simulink model "crazyflie_ponti"  (R2018b)
settings: Solver=FixedStepDiscrete  StartTime=0.0  StopTime=25  FixedStep=0.01  RelTol=1e-3
values from neighbouring files (symbols this model uses):
  gamma = 0.98    [Jonaz.mat]
  K = [-135.279629651 -135.279629543 135.279629485 135.279629377 -135.330448309 135.330448003 135.330448111 -135.330448202 -58.4203591404 -58.4203590939 58.420359069 58.4203590225 ... (20 elements, 4x5)]    [Jonaz.mat]    (also in LQRGain.mat)
undefined symbols (not defined in the file or in its folder): DiscIntNeverNeededParam
libraries: simulink x1
settings Model: PauseTimes=7  Creator=Zrean  LastModifiedBy=Jonas
settings OptimizationCC: DefaultParameterBehavior=Inlined  UseDivisionForNetSlopeComputation=on  UseFloatMulNetSlope=on  UseSpecifiedMinMax=on  InlineInvariantSignals=on  PassReuseOutputArgsAs=Individual arguments  ZeroExternalMemoryAtStartup=off  ZeroInternalMemoryAtStartup=off  NoFixptDivByZeroProtection=on  EfficientFloat2IntCast=on  LifeSpan=1
settings DebuggingCC: AlgebraicLoopMsg=error  ParameterTunabilityLossMsg=error
settings HardwareCC: ProdBitPerPointer=32  ProdBitPerSizeT=32  ProdBitPerPtrDiffT=32  ProdLargestAtomicInteger=Long  ProdLargestAtomicFloat=Double  ProdWordSize=32  ProdHWDeviceType=ARM Compatible->ARM Cortex
settings SFSimCC: SimUseLocalCustomCode=off  MATLABDynamicMemAlloc=off
settings RTWCC: SystemTargetFile=ert.tlc  GenCodeOnly=on  TemplateMakefile=ert_default_tmf  GenerateReport=on  RTWUseLocalCustomCode=off  BuildConfiguration=Faster Runs  IncludeHyperlinkInReport=on  LaunchReport=on  GenerateTraceInfo=on  GenerateTraceReport=on  GenerateTraceReportSl=on  GenerateTraceReportSf=on  GenerateTraceReportEml=on  GenerateCodeMetricsReport=on
settings CodeAppCC: ForceParamTrailComments=on  IgnoreCustomStorageClasses=off  OperatorAnnotations=on  SimulinkDataObjDesc=on  SFDataObjDesc=on  MATLABFcnDesc=on  CustomSymbolStrGlobalVar=rt$N$M  CustomSymbolStrType=$N$M  CustomSymbolStrFcn=$N$M$F  CustomSymbolStrMacro=$N$M  InsertBlockDesc=on  StateflowObjectComments=on  MATLABSourceComments=on
settings ERTTargetCC: TargetLangStandard=C99 (ISO)  MultiwordLength=2048  CombineSignalStateStructs=on  SuppressErrorStatus=on  SupportAbsoluteTime=off  SupportNonFinite=off  SupportComplex=off  InlinedParameterPlacement=NonHierarchical  ERTCustomFileTemplate=crazyflie_wrapper.tlc  ERTFilePackagingFormat=CompactWithDataFile
settings SimscapeCC: SimscapeNormalizeSystem=off

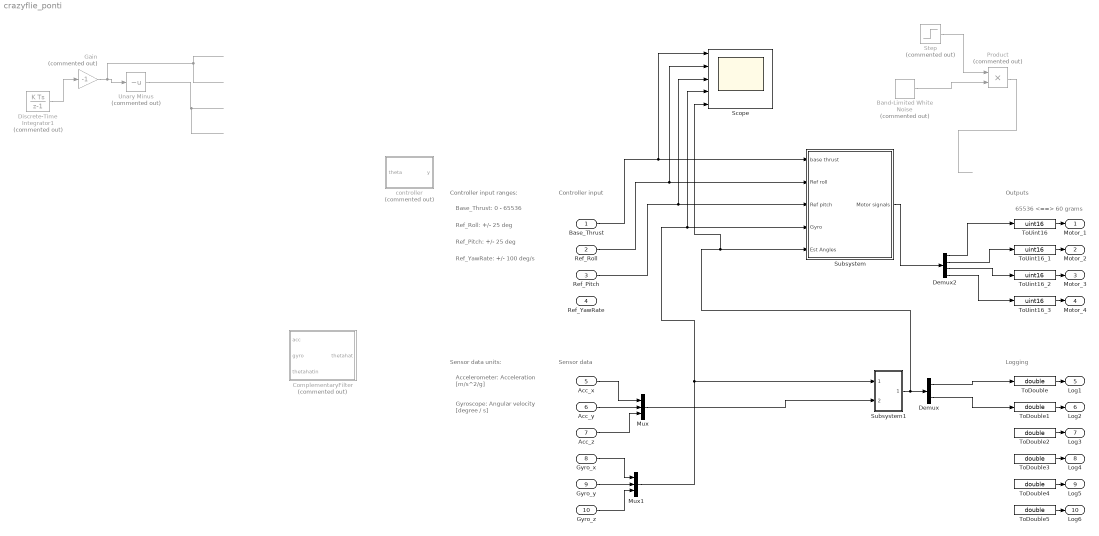
== system crazyflie_ponti ==
  note: 65536 <==> 60 grams
  note: Logging
  note: Outputs
  note: Sensor data
  note: Controller input
  note: Ref_Roll: +/- 25 deg
  note: Base_Thrust: 0 - 65536
  note: Ref_Pitch: +/- 25 deg
  note: Ref_YawRate: +/- 100 deg/s
  note: Controller input ranges:
  note: Gyroscope:
      | Angular velocity [degree / s]
  note: Accelerometer:
      | Acceleration [m/s^2/g]
  note: Sensor data units:
  Base_Thrust : Inport  OutDataTypeStr=double
  Ref_Roll : Inport  Port=2  OutDataTypeStr=double
  Ref_Pitch : Inport  Port=3  OutDataTypeStr=double
  Ref_YawRate : Inport  Port=4  OutDataTypeStr=double
  Acc_x : Inport  Port=5  OutDataTypeStr=double  PortDimensions=1
  Acc_y : Inport  Port=6  OutDataTypeStr=double  PortDimensions=1
  Acc_z : Inport  Port=7  OutDataTypeStr=double  PortDimensions=1
  Gyro_x : Inport  Port=8  OutDataTypeStr=double  PortDimensions=1
  Gyro_y : Inport  Port=9  OutDataTypeStr=double  PortDimensions=1
  Gyro_z : Inport  Port=10  OutDataTypeStr=double  PortDimensions=1
  Band-Limited White Noise : simulink/Sources/Band-Limited White Noise  Commented=on  Cov=[10]  Ts=2  seed=[23341]
  "ComplementaryFilter " : MATLAB Function  Commented=on  TreatAsAtomicUnit=on
  Demux : Demux  Outputs=2
  Demux2 : Demux
  Discrete-Time Integrator1 : DiscreteIntegrator  Commented=on  SampleTime=-1  ICPrevOutput=DiscIntNeverNeededParam  ICPrevScaledInput=DiscIntNeverNeededParam
  Gain : Gain  Commented=on  Gain=-1
  Mux : Mux  Inputs=3
  Mux1 : Mux  Inputs=3
  Product : Product  Commented=on
  Scope : Scope  NumInputPorts=5
  Step : Step  Commented=on  Time=2  After=0  SampleTime=0
  Subsystem : Subsystem
  Subsystem1 : Subsystem
  ToDouble{,1..5} (6 alike) : DataTypeConversion  OutDataTypeStr=double  SaturateOnIntegerOverflow=on
  ToUint16 : DataTypeConversion  OutDataTypeStr=uint16  SaturateOnIntegerOverflow=on
  ToUint16_1 : DataTypeConversion  OutDataTypeStr=uint16  SaturateOnIntegerOverflow=on
  ToUint16_2 : DataTypeConversion  OutDataTypeStr=uint16  SaturateOnIntegerOverflow=on
  ToUint16_3 : DataTypeConversion  OutDataTypeStr=uint16  SaturateOnIntegerOverflow=on
  Unary Minus : UnaryMinus  Commented=on
  controller : MATLAB Function  Commented=on  TreatAsAtomicUnit=on
  Motor_1 : Outport  OutDataTypeStr=uint16  LockScale=on
  Motor_2 : Outport  Port=2  OutDataTypeStr=uint16  LockScale=on
  Motor_3 : Outport  Port=3  OutDataTypeStr=uint16  LockScale=on
  Motor_4 : Outport  Port=4  OutDataTypeStr=uint16  LockScale=on
  Log1 : Outport  Port=5  OutDataTypeStr=double
  Log2 : Outport  Port=6  OutDataTypeStr=double
  Log3 : Outport  Port=7  OutDataTypeStr=double
  Log4 : Outport  Port=8  OutDataTypeStr=double
  Log5 : Outport  Port=9  OutDataTypeStr=double
  Log6 : Outport  Port=10  OutDataTypeStr=double
  wires:
  ToUint16/1 -> Motor_1/1
  ToUint16_1/1 -> Motor_2/1
  ToUint16_2/1 -> Motor_3/1
  ToUint16_3/1 -> Motor_4/1
  ToDouble/1 -> Log1/1
  ToDouble1/1 -> Log2/1
  ToDouble2/1 -> Log3/1
  ToDouble3/1 -> Log4/1
  ToDouble4/1 -> Log5/1
  ToDouble5/1 -> Log6/1
  Acc_z/1 -> Mux/3
  Acc_x/1 -> Mux/1
  Acc_y/1 -> Mux/2
  Gyro_z/1 -> Mux1/3
  Mux1/1 -> Scope/4, Subsystem/4(Gyro), Subsystem1/1(Gyro)
  Gyro_x/1 -> Mux1/1
  Gain/1 -> Unary Minus/1
  Unary Minus/1 -> ?
  Discrete-Time Integrator1/1 -> Gain/1
  Demux2/2 -> ToUint16_1/1
  Demux2/3 -> ToUint16_2/1
  Demux2/4 -> ToUint16_3/1
  Gyro_y/1 -> Mux1/2
  Base_Thrust/1 -> Scope/1, Subsystem/1(base thrust)
  Ref_Roll/1 -> Scope/2, Subsystem/2(Ref roll)
  Ref_Pitch/1 -> Scope/3, Subsystem/3(Ref pitch)
  Subsystem/1("Motor signals ") -> Demux2/1
  Mux/1 -> Subsystem1/2(Acc)
  Subsystem1/1(Out1) -> Demux/1, Scope/5, Subsystem/5(Est Angles)
  Demux2/1 -> ToUint16/1
  Step/1 -> Product/1
  Band-Limited White Noise/1 -> Product/2
  Product/1 -> ?
  Demux/1 -> ToDouble/1
  Demux/2 -> ToDouble1/1

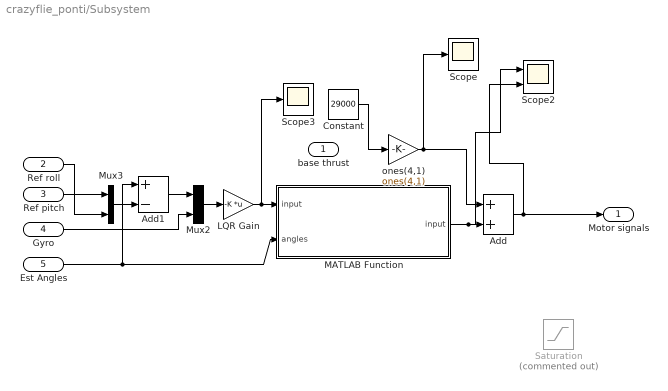
== system crazyflie_ponti/Subsystem ==
  base thrust : Inport
  Ref roll : Inport  Port=2
  Ref pitch : Inport  Port=3
  Gyro : Inport  Port=4
  Est Angles : Inport  Port=5
  Add : Sum
  Add1 : Sum  Inputs=+-
  Constant : Constant  Value=29000
  LQR Gain : Gain  Gain=-K  Multiplication=Matrix(K*u)
  MATLAB Function : MATLAB Function  TreatAsAtomicUnit=on
  Mux2 : Mux  Inputs=2
  Mux3 : Mux  Inputs=2
  Saturation : Saturate  Commented=on  UpperLimit=65536  LowerLimit=0
  Scope : Scope
  Scope2 : Scope  NumInputPorts=2
  Scope3 : Scope
  ones(4,1) : Gain  Gain=ones(4,1)
  "Motor signals " : Outport
  wires:
  Add/1 -> "Motor signals "/1, Scope2/2
  Mux2/1 -> LQR Gain/1
  ones(4,1)/1 -> Scope/1, Add/1
  LQR Gain/1 -> Scope3/1, MATLAB Function/1("input ")
  Ref pitch/1 -> Mux3/2
  Ref roll/1 -> Mux3/1
  Add1/1 -> Mux2/1
  MATLAB Function/1(input) -> Scope2/1, Add/2
  Gyro/1 -> Mux2/2
  Est Angles/1 -> Add1/1, MATLAB Function/2(angles)
  Mux3/1 -> Add1/2
  Constant/1 -> ones(4,1)/1

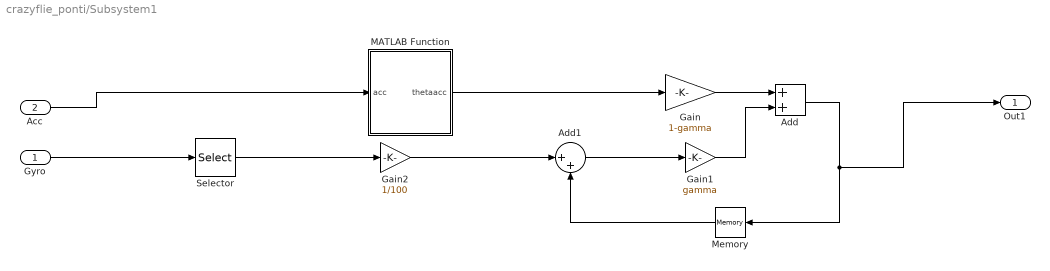
== system crazyflie_ponti/Subsystem1 ==
  Gyro : Inport
  Acc : Inport  Port=2
  Add : Sum
  Add1 : Sum  Inputs=|++
  Gain : Gain  Gain=1-gamma
  Gain1 : Gain  Gain=gamma
  Gain2 : Gain  Gain=1/100
  MATLAB Function : MATLAB Function  TreatAsAtomicUnit=on
  Memory : Memory  InitialCondition=[0 0]
  Selector : Selector  InputPortWidth=3  IndexOptions=Index vector (dialog)  Indices=[1 2]  OutputSizes=1
  Out1 : Outport
  wires:
  Acc/1 -> MATLAB Function/1(acc)
  Gyro/1 -> Selector/1
  MATLAB Function/1(thetaacc) -> Gain/1
  Gain/1 -> Add/1
  Gain1/1 -> Add/2
  Add1/1 -> Gain1/1
  Gain2/1 -> Add1/1
  Selector/1 -> Gain2/1
  Memory/1 -> Add1/2
  Add/1 -> Out1/1, Memory/1

== matlab function crazyflie_ponti/controller ==
  data: theta input; y output
function y = fcn(theta)
motors = zeros(4,1);
K=65536*0.2;
threshold = 0.02;
if theta(1)<-threshold
    motors(3) = motors(3) + K*abs(theta(1));
    motors(2) = motors(2) + K*abs(theta(1));
elseif theta(1)>threshold
    motors(1) = motors(1) + K*abs(theta(1));
    motors(4) = motors(4) + K*abs(theta(1));
end

if theta(2)<-threshold
    motors(4) = motors(4) + K*abs(theta(2));
    motors(3) = motors(3) + K*abs(theta(2));
elseif theta(2)>threshold
    motors(1) = motors(1) + K*abs(theta(2));
    motors(2) = motors(2) + K*abs(theta(2));
end
y = motors;

== matlab function crazyflie_ponti/Subsystem/MATLAB Function ==
  data: input input; input output; angles input
function input = TurnOffIfUpsideDown(input, angles)

if isnan(input)
    input = zeros(4,1);
end
a = input;

threshold = 60;
if ((abs(angles(1))>threshold || abs(angles(2)>threshold)))
   a = zeros(4,1);
end
input = a;

== matlab function crazyflie_ponti/Subsystem1/MATLAB Function ==
  data: acc input; thetaacc output
function thetaacc = AccAngles(acc)

acc = acc./norm(acc);

rollacc = (180/pi)*atan2(acc(2),acc(3));
pitchacc = (180/pi)*atan2(-acc(1), sqrt(acc(2)^2+acc(3)^2));

thetaacc = [rollacc;pitchacc];

== matlab function crazyflie_ponti/ComplementaryFilter  ==
  data: acc input; gyro input; thetahat output; thetahatin input
function thetahat    = FusionFilter(acc, gyro, thetahatin)
h = 1/100;
% alpha = .001;
% gamma = alpha/(h+alpha);
gamma = 0.98;

acc = acc./norm(acc);

% rollacc = atan2(acc(2),acc(3));
% pitchacc = atan2(-acc(1), sqrt(acc(2)^2+acc(3)^2));
% %accout = [pitchacc;rollacc];
% thetahat1 = thetahatin + h*[gyro(2); gyro(1); 0];
% thetahat = (1-gamma)*[pitchacc;rollacc;0]+gamma*thetahat1;

rollacc = (180/pi)*atan2(acc(2),acc(3));
pitchacc = (180/pi)*atan2(-acc(1), sqrt(acc(2)^2+acc(3)^2));
%accout = [pitchacc;rollacc];
thetahat1 = thetahatin + h*[gyro(1); gyro(2)];
thetahat = (1-gamma)*[rollacc;pitchacc]+gamma*thetahat1;
